simulink model "ilcModel"  (R2021b)
settings: Solver=VariableStepAuto  StartTime=0.0  StopTime=10.0  RelTol=1e-3
libraries: vrlib x2, shared6dof x1, dspmtrx3 x1, sldrtlib x1
settings Model: Creator=josep  LastModifiedBy=josep

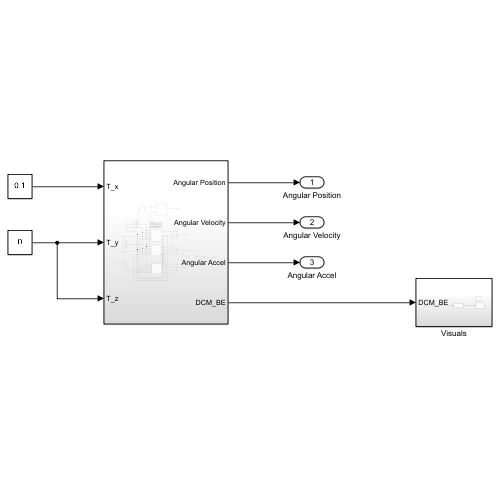
[thumbnail: Simulink's stored preview of the top-level diagram]
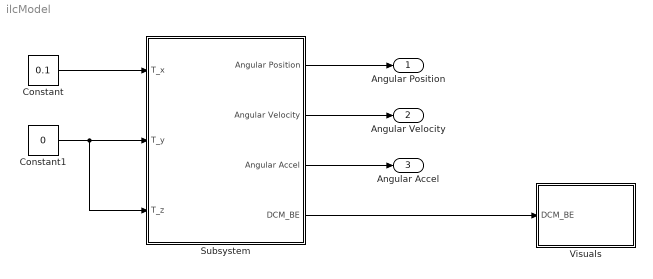
== system ilcModel ==
  Constant : Constant  Value=0.1
  Constant1 : Constant  Value=0
  Subsystem : Subsystem
  Visuals : Subsystem
  Angular Position : Outport
  Angular Velocity : Outport  Port=2
  Angular Accel : Outport  Port=3
  wires:
  Subsystem/1(Angular Position) -> Angular Position/1
  Subsystem/2(Angular Velocity) -> Angular Velocity/1
  Subsystem/3(Angular Accel) -> Angular Accel/1
  Subsystem/4(DCM_BE) -> Visuals/1(DCM_BE)
  Constant/1 -> Subsystem/1(T_x)
  Constant1/1 -> Subsystem/3(T_z), Subsystem/2(T_y)

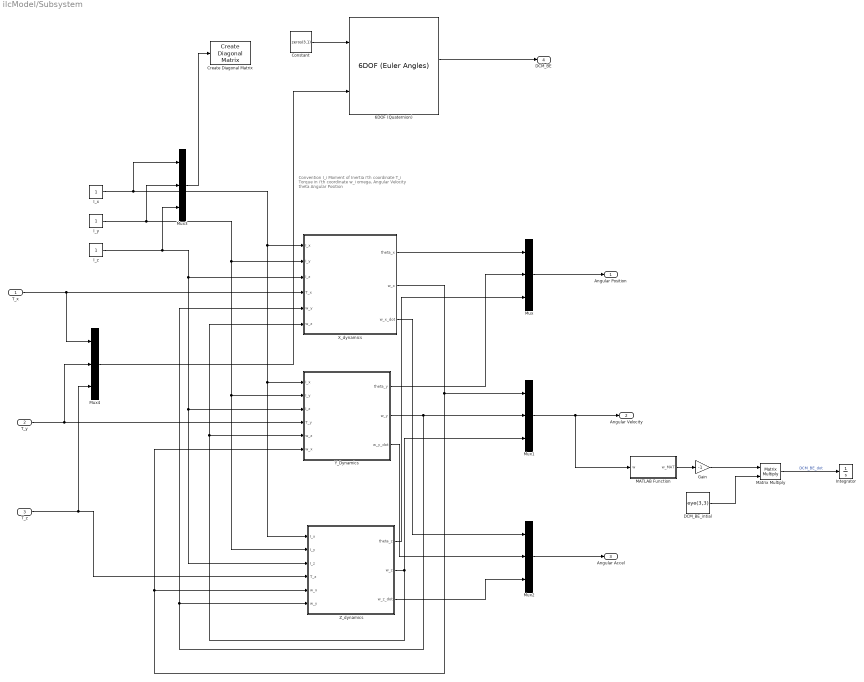
== system ilcModel/Subsystem ==
  note: Convention
      |
      | I_i
      | Moment of Inertia i'th coordinate
      |
      | T_i
      | Torque in i'th coordinate
      |
      | w_i
      | omega, Angular Velocity
      |
      | theta
      | Angular Position
  T_x : Inport
  T_y : Inport  Port=2
  T_z : Inport  Port=3
  6DOF (Quaternion) : shared6dof/6DOF (Euler Angles)  units=Metric (MKS)  mtype=Fixed  rep=Quaternion  xme_0=[0 0 0]  Vm_0=[0 0 0]  eul_0=[0 0 0]  pm_0=[0 0 0]  mass_0=1.0  mass_e=0.5  mass_f=2.0  inertia=eye(3)  inertia_e=eye(3)  inertia_f=2*eye(3)  k_quat=1.0  vre_flag=on  abi_flag=off  aMode=0  xme_statename=''  Vm_statename=''  eul_statename=''  quat_statename=''  pm_statename=''  mass_statename=''
      settings: SourceProductBaseCode=AE,PW,DR,MT,UV,VE
  Constant : Constant  Value=zeros(3,1)
  Create Diagonal Matrix : dspmtrx3/Create Diagonal Matrix
      settings: SourceProductBaseCode=DS
  DCM_BE_intial : Constant  Value=eye(3,3)
  Gain : Gain  Gain=-1
  I_x : Constant
  I_y : Constant
  I_z : Constant
  Integrator : Integrator
  MATLAB Function : MATLAB Function  TreatAsAtomicUnit=on
  Matrix Multiply : Product  Multiplication=Matrix(*)
  Mux{,1..4} (5 alike) : Mux  Inputs=3
  X_dynamics : Subsystem
  Y_Dynamics : Subsystem
  Z_dynamics : Subsystem
  Angular Position : Outport
  Angular Velocity : Outport  Port=2
  Angular Accel : Outport  Port=3
  DCM_BE : Outport  Port=4
  wires:
  Z_dynamics/1(theta_z) -> Mux/3
  Y_Dynamics/2(w_y) -> Mux1/2, Z_dynamics/6(w_y), X_dynamics/5(w_y)
  T_z/1 -> Mux4/3, Z_dynamics/4(T_z)
  X_dynamics/2(w_x) -> Mux1/1, Z_dynamics/5(w_x), Y_Dynamics/6(w_x)
  I_x/1 -> Mux3/1, Z_dynamics/1(I_x), Y_Dynamics/1(I_x), X_dynamics/1(I_x)
  I_z/1 -> Mux3/3, Z_dynamics/3(I_z), Y_Dynamics/3(I_z), X_dynamics/3(I_z)
  T_y/1 -> Mux4/2, Y_Dynamics/4(T_y)
  I_y/1 -> Mux3/2, Z_dynamics/2(I_y), Y_Dynamics/2(I_y), X_dynamics/2(I_y)
  Z_dynamics/2(w_z) -> Y_Dynamics/5(w_z), X_dynamics/6(w_z), Mux1/3
  Mux2/1 -> Angular Accel/1
  T_x/1 -> Mux4/1, X_dynamics/4(T_x)
  Y_Dynamics/3(w_y_dot) -> Mux2/2
  Y_Dynamics/1(theta_y) -> Mux/2
  Z_dynamics/3(w_z_dot) -> Mux2/3
  Mux/1 -> Angular Position/1
  X_dynamics/1(theta_x) -> Mux/1
  X_dynamics/3(w_x_dot) -> Mux2/1
  Mux1/1 -> MATLAB Function/1(w), Angular Velocity/1
  MATLAB Function/1(w_MAT) -> Gain/1
  Gain/1 -> Matrix Multiply/1
  DCM_BE_intial/1 -> Matrix Multiply/2
  Matrix Multiply/1 -> Integrator/1  "DCM_BE_dot"
  Mux3/1 -> Create Diagonal Matrix/1
  Mux4/1 -> 6DOF (Quaternion)/2
  Constant/1 -> 6DOF (Quaternion)/1
  6DOF (Quaternion)/4 -> DCM_BE/1

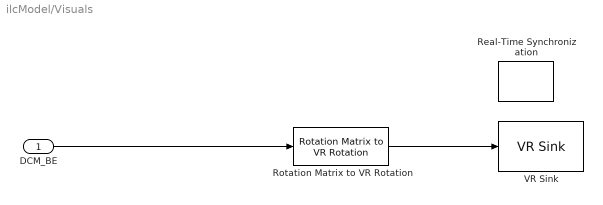
== system ilcModel/Visuals ==
  DCM_BE : Inport
  Real-Time Synchronization : sldrtlib/Real-Time Synchronization  SampleTime=0.1  MaxMissedTicks=10  ShowMissedTicks=off  YieldWhenWaiting=off
  Rotation Matrix to VR Rotation : vrlib/Utilities/Rotation Matrix to VR Rotation  maxzero=1e-12
      settings: SourceProductBaseCode=SL
  VR Sink : vrlib/VR Sink  InstantiateOnLoad=on  SampleTime=-1  ViewEnable=on  RemoteChange=off  RemoteView=off  FieldsWritten=CubeSat.rotation.4.1.1.double  WorldFileName=VRSinkFiles\ILCSimulink\CubeSat.x3d  AutoView=off  VideoDimensions=[]  AllowVariableSize=off  FigureProperties="{'Position', 'Name', 'Viewpoint', 'CameraBound', 'CameraDirection', 'CameraPosition', 'CameraUpVector', 'ZoomFactor', 'Antialiasing', 'Headlight', 'Lighting', 'NavPanel', 'Sound', 'StatusBar', 'Stereo3D', 'Stereo3DCameraOffset', 'Stereo3DHIT', 'ToolBar', 'Textures', 'Transparency', 'Triad', 'Wireframe', 'NavZones', 'NavMode', 'NavSpeed', 'CaptureFileFormat', 'CaptureFileName', 'Record2DCompressMethod', 'Record2DCompressQuality', 'Record2D', 'Record2DFileName', 'Record2DFPS'; [1.1130000000000000e+03   3.1020000000000005e+02   5.7600000000000000e+02   3.5000000000000000e+02], '', '', 'on', [0.0000000000000000e+00   3.1410759078128292e-02  -9.9950656036573160e-01], [0.0000000000000000e+00   0.0000000000000000e+00   5.8497421741485596e+00], [0.0000000000000000e+00   9.9950656036573160e-01   3.1410759078128292e-02], [1.0000000000000000e+00], 'on', 'on', 'on', 'halfbar', 'on', 'on', 'off', [1.0000000149011612e-01], [0.0000000000000000e+00], 'on', 'on', 'on', 'none', 'off', 'off', 'fly', 'normal', 'tif', '%f_anim_%n.tif', 'auto', [7.5000000000000000e+01], 'off', '%f_anim_%n.avi', 'auto'}"
  wires:
  DCM_BE/1 -> Rotation Matrix to VR Rotation/1
  Rotation Matrix to VR Rotation/1 -> VR Sink/1

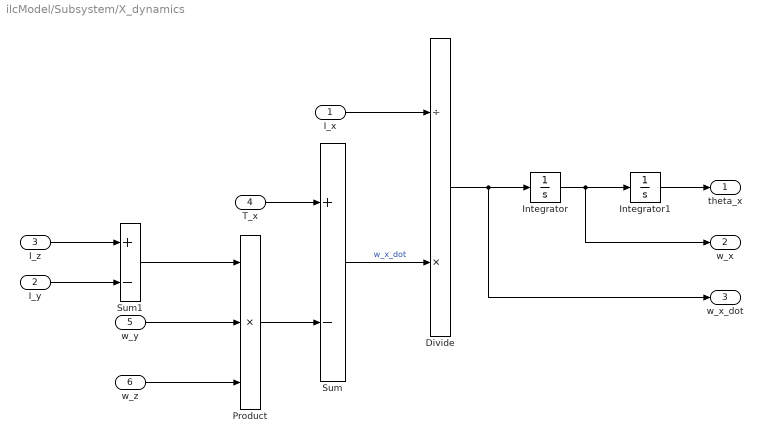
== system ilcModel/Subsystem/X_dynamics ==
  I_x : Inport
  I_y : Inport  Port=2
  I_z : Inport  Port=3
  T_x : Inport  Port=4
  w_y : Inport  Port=5
  w_z : Inport  Port=6
  Divide : Product  Inputs=/*
  Integrator : Integrator
  Integrator1 : Integrator
  Product : Product  Inputs=3
  Sum : Sum  Inputs=+-
  Sum1 : Sum  Inputs=+-
  theta_x : Outport
  w_x : Outport  Port=2
  w_x_dot : Outport  Port=3
  wires:
  Divide/1 -> Integrator/1, w_x_dot/1
  T_x/1 -> Sum/1
  Product/1 -> Sum/2
  w_z/1 -> Product/3
  Integrator/1 -> Integrator1/1, w_x/1
  Sum/1 -> Divide/2  "w_x_dot"
  Sum1/1 -> Product/1
  I_z/1 -> Sum1/1
  I_y/1 -> Sum1/2
  I_x/1 -> Divide/1
  Integrator1/1 -> theta_x/1
  w_y/1 -> Product/2

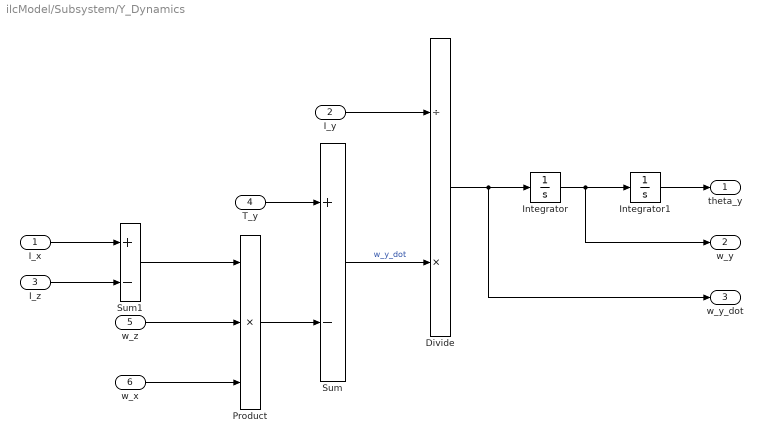
== system ilcModel/Subsystem/Y_Dynamics ==
  I_x : Inport
  I_y : Inport  Port=2
  I_z : Inport  Port=3
  T_y : Inport  Port=4
  w_z : Inport  Port=5
  w_x : Inport  Port=6
  Divide : Product  Inputs=/*
  Integrator : Integrator
  Integrator1 : Integrator
  Product : Product  Inputs=3
  Sum : Sum  Inputs=+-
  Sum1 : Sum  Inputs=+-
  theta_y : Outport
  w_y : Outport  Port=2
  w_y_dot : Outport  Port=3
  wires:
  Divide/1 -> Integrator/1, w_y_dot/1
  T_y/1 -> Sum/1
  Product/1 -> Sum/2
  w_x/1 -> Product/3
  Integrator/1 -> Integrator1/1, w_y/1
  Sum/1 -> Divide/2  "w_y_dot"
  Sum1/1 -> Product/1
  I_x/1 -> Sum1/1
  I_z/1 -> Sum1/2
  I_y/1 -> Divide/1
  Integrator1/1 -> theta_y/1
  w_z/1 -> Product/2

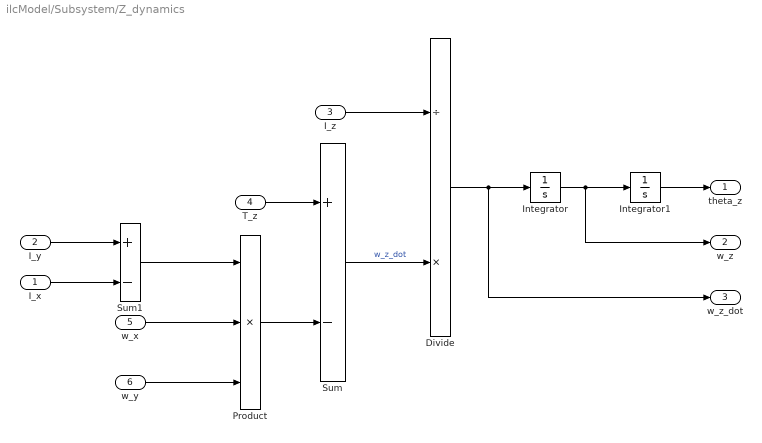
== system ilcModel/Subsystem/Z_dynamics ==
  I_x : Inport
  I_y : Inport  Port=2
  I_z : Inport  Port=3
  T_z : Inport  Port=4
  w_x : Inport  Port=5
  w_y : Inport  Port=6
  Divide : Product  Inputs=/*
  Integrator : Integrator
  Integrator1 : Integrator
  Product : Product  Inputs=3
  Sum : Sum  Inputs=+-
  Sum1 : Sum  Inputs=+-
  theta_z : Outport
  w_z : Outport  Port=2
  w_z_dot : Outport  Port=3
  wires:
  Divide/1 -> Integrator/1, w_z_dot/1
  T_z/1 -> Sum/1
  Product/1 -> Sum/2
  w_y/1 -> Product/3
  Integrator/1 -> Integrator1/1, w_z/1
  Sum/1 -> Divide/2  "w_z_dot"
  Sum1/1 -> Product/1
  I_y/1 -> Sum1/1
  I_x/1 -> Sum1/2
  I_z/1 -> Divide/1
  Integrator1/1 -> theta_z/1
  w_x/1 -> Product/2

== matlab function ilcModel/Subsystem/MATLAB Function ==
  data: w input; w_MAT output
function w_MAT= crossop(w)
% Converts input columne vector into cross product matrix
w_MAT = [ 0   -w(3) w(2)
          w(3) 0   -w(1)
         -w(2) w(1) 0  ];
